simulink model "thermal_model_of_analysis"  (R2017a)
settings: Solver=VariableStepAuto  StartTime=0.0  StopTime=1  RelTol=1e-3
values from neighbouring files (symbols this model uses):
  R_tim = 1.5    [plot_code.m]
  Rth_heatsink = 0.01*i    [plot_code.m]
  Rth_jc = 0.5    [plot_code.m]
  Rth_pcb = 4.5    [plot_code.m]
libraries: fl_lib x11, nesl_utility x4
settings Model: Creator=Caner  LastModifiedBy=Caner

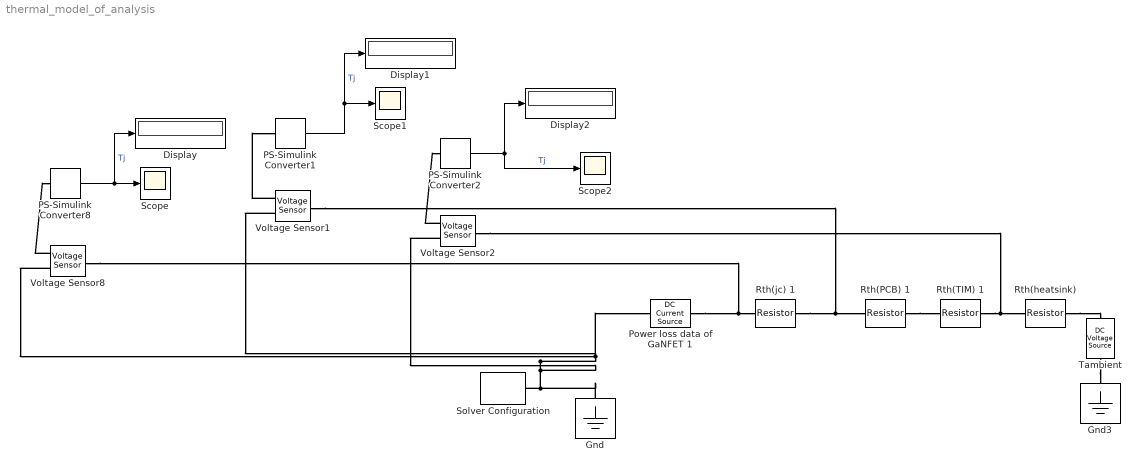
== system thermal_model_of_analysis ==
  Display : Display
  Display1 : Display
  Display2 : Display
  Gnd : fl_lib/Electrical/Electrical Elements/Electrical Reference
  Gnd3 : fl_lib/Electrical/Electrical Elements/Electrical Reference
  PS-Simulink Converter1 : nesl_utility/PS-Simulink Converter  PhysicalDomain=network_engine_domain  SubClassName=ps_output  LeftPortType=input  RightPortType=output  PseudoPeriodic=off  Frequencies=[]  Unit=1  AffineConversion=off
  PS-Simulink Converter2 : nesl_utility/PS-Simulink Converter  PhysicalDomain=network_engine_domain  SubClassName=ps_output  LeftPortType=input  RightPortType=output  PseudoPeriodic=off  Frequencies=[]  Unit=1  AffineConversion=off
  PS-Simulink Converter8 : nesl_utility/PS-Simulink Converter  PhysicalDomain=network_engine_domain  SubClassName=ps_output  LeftPortType=input  RightPortType=output  PseudoPeriodic=off  Frequencies=[]  Unit=1  AffineConversion=off
  Power loss data of GaNFET 1 : fl_lib/Electrical/Electrical Sources/DC Current Source  i0=Power_loss A
      settings: SourceProductName=Simscape  SourceProductBaseCode=SS
  Rth(PCB) 1 : fl_lib/Electrical/Electrical Elements/Resistor  R=Rth_pcb Ohm  i_specify=off  i_priority=High  i=0 A  i_nominal_specify=off  i_nominal_unit=A  i_nominal_value=1  v_specify=off  v_priority=High  v=0 V  v_nominal_specify=off  v_nominal_unit=V  v_nominal_value=1
  Rth(TIM) 1 : fl_lib/Electrical/Electrical Elements/Resistor  R=R_tim Ohm  i_specify=off  i_priority=High  i=0 A  i_nominal_specify=off  i_nominal_unit=A  i_nominal_value=1  v_specify=off  v_priority=High  v=0 V  v_nominal_specify=off  v_nominal_unit=V  v_nominal_value=1
  "Rth(heatsink) " : fl_lib/Electrical/Electrical Elements/Resistor  R=Rth_heatsink Ohm  i_specify=off  i_priority=High  i=0 A  i_nominal_specify=off  i_nominal_unit=A  i_nominal_value=1  v_specify=off  v_priority=High  v=0 V  v_nominal_specify=off  v_nominal_unit=V  v_nominal_value=1
  Rth(jc) 1 : fl_lib/Electrical/Electrical Elements/Resistor  R=Rth_jc Ohm  i_specify=off  i_priority=High  i=0 A  i_nominal_specify=off  i_nominal_unit=A  i_nominal_value=1  v_specify=off  v_priority=High  v=0 V  v_nominal_specify=off  v_nominal_unit=V  v_nominal_value=1
  Scope : Scope
  Scope1 : Scope
  Scope2 : Scope
  Solver Configuration : nesl_utility/Solver Configuration  PhysicalDomain=network_engine_domain  SubClassName=solver  LeftPortType=input  RightPortType=generic  Accelerate=off  Tones=[]  Harmonics=[]  SimulateNoise=off  Profile=off  UseLocalSampling=off  EnableSwitchedLinearOptims=on  FrequencyDomain=off  UseCCode=off  RelTol=0.001  AbsTol=1e-06  MinStep=1e-09  ToWorkspace=off  RevertToSquareIcSolve=off  NumHomotopyIterations=100  PhasorMode=off  PhasorModeNumHarmonics=1  OverrideAbsTol=off  DoDC=off  ResidualTolerance=1e-09  UseLocalSolver=off  LocalSolverChoice=NE_BACKWARD_EULER_ADVANCER  LocalSolverSampleTime=0.001  DoFixedCost=off  MaxNonlinIter=3  MaxModeIter=2  LinearAlgebra=Sparse  DelaysMemoryBudget=1024  AutomaticFiltering=on  FilteringTimeConstant=0.001
  Tambient : fl_lib/Electrical/Electrical Sources/DC Voltage Source  v0=T_ambient V
  Voltage Sensor1 : fl_lib/Electrical/Electrical Sensors/Voltage Sensor
  Voltage Sensor2 : fl_lib/Electrical/Electrical Sensors/Voltage Sensor
  Voltage Sensor8 : fl_lib/Electrical/Electrical Sensors/Voltage Sensor
  wires:
  PS-Simulink Converter8/1 -> Display/1, Scope/1  "Tj"
  PS-Simulink Converter1/1 -> Display1/1, Scope1/1  "Tj"
  PS-Simulink Converter2/1 -> Display2/1, Scope2/1  "Tj"
  connections:
  Solver Configuration/RConn1 -- Voltage Sensor2/RConn2 -- Voltage Sensor1/RConn2 -- Power loss data of GaNFET 1/RConn1 -- Voltage Sensor8/RConn2 -- Gnd/LConn1
  Rth(TIM) 1/RConn1 -- Voltage Sensor2/LConn1 -- "Rth(heatsink) "/LConn1
  Rth(jc) 1/RConn1 -- Voltage Sensor1/LConn1 -- Rth(PCB) 1/LConn1
  Tambient/RConn1 -- Gnd3/LConn1
  "Rth(heatsink) "/RConn1 -- Tambient/LConn1
  Voltage Sensor8/RConn1 -- PS-Simulink Converter8/LConn1
  Power loss data of GaNFET 1/LConn1 -- Voltage Sensor8/LConn1 -- Rth(jc) 1/LConn1
  Rth(PCB) 1/RConn1 -- Rth(TIM) 1/LConn1
  Voltage Sensor1/RConn1 -- PS-Simulink Converter1/LConn1
  Voltage Sensor2/RConn1 -- PS-Simulink Converter2/LConn1
